simulink model "Dougherty1968_Linear"  (R2022b)
settings: Solver=VariableStepAuto  StartTime=0.0  StopTime=5000  RelTol=1e-3
model workspace (MAT data in the model file):
  Ix = 1000
  Iy = 1000
  Iz = 1000
  K_i = 1150
  K_p = 25
  T_c = 1
  frequency_multiplier = 10000
  h = 150
  k_phi = 50
  offset = 0.611
  omega_0 = 0.000727
  phi_0 = 0.0175
  phi_dot_0 = 0
  psi_0 = 0
  psi_dot_0 = 0
  tau = 25
libraries: simulink x2
settings Model: Creator=Kirtan  LastModifiedBy=Kirtan

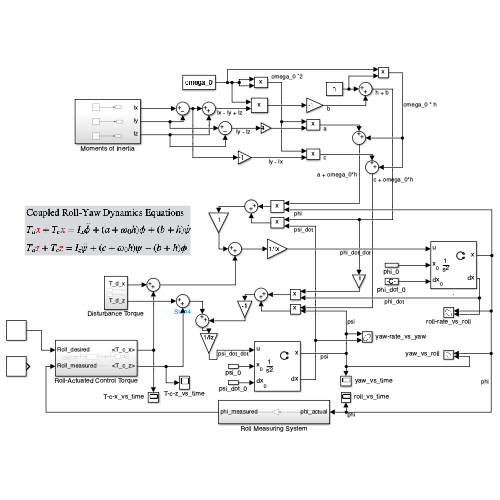
[thumbnail: Simulink's stored preview of the top-level diagram]
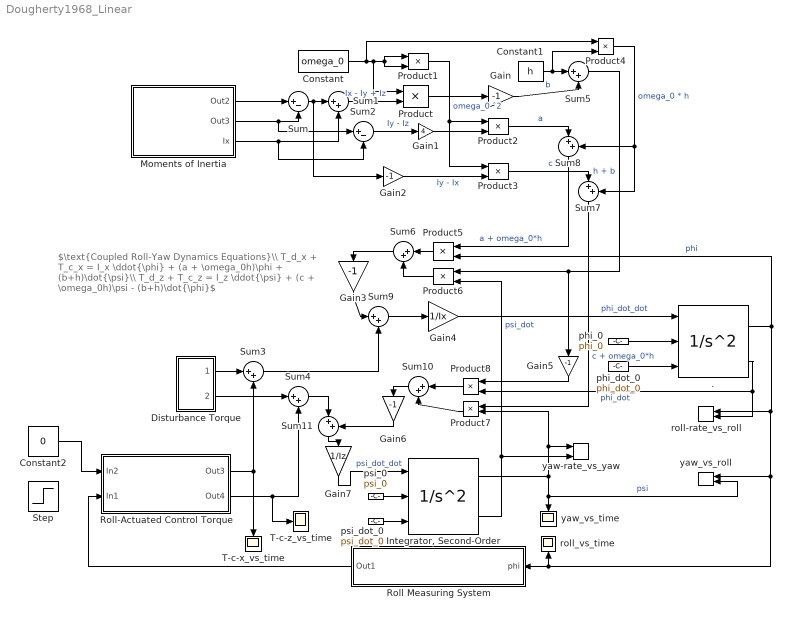
== system Dougherty1968_Linear ==
  note: $\text{Coupled Roll-Yaw Dynamics Equations}\\ T_d_x + T_c_x = I_x \ddot{\phi} + (a + \omega_0h)\phi + (b+h)\dot{\psi}\\ T_d_z + T_c_z = I_z \ddot{\psi} + (c + \omega_0h)\psi - (b+h)\dot{\phi}$
  . : SecondOrderIntegrator  ICSourceX=external  ICX=0.0175  WrapX=on  ICSourceDXDT=external
  Constant : Constant  Value=omega_0
  Constant1 : Constant  Value=h
  Constant2 : Constant  Value=0
  Disturbance Torque : Subsystem
  Gain{,2..3,5..6} (5 alike) : Gain  Gain=-1
  Gain1 : Gain  Gain=4
  Gain4 : Gain  Gain=1/Ix
  Gain7 : Gain  Gain=1/Iz
  "Integrator, Second-Order" : SecondOrderIntegrator  ICSourceX=external  ICX=0  WrapX=on  ICSourceDXDT=external
  Moments of Inertia : Subsystem
  Product{,1..8} (9 alike) : Product
  Roll Measuring System : Subsystem
  Roll-Actuated Control Torque : Subsystem
  Step : Step  After=0.5  SampleTime=0
  Sum : Sum  Inputs=|+-
  Sum{1,3..11} (10 alike) : Sum  Inputs=|++
  Sum2 : Sum  Inputs=|+-
  T-c-x_vs_time : Scope
  T-c-z_vs_time : Scope
  phi_0 : Constant  Value=phi_0
  phi_dot_0 : Constant  Value=phi_dot_0
  psi_0 : Constant  Value=psi_0
  psi_dot_0 : Constant  Value=psi_dot_0
  roll-rate_vs_roll : Record  FileSettingsInternal="{\"entries\":[{\"content\":{\"excelSettings\":{\"content\":{},\"type\":\"Streamout.ExcelSettings\"}},\"type\":\"Streamout.FileSettingStorage\",\"uuid\":\"38b1782c-b750-4221-bec9-1b26ef69e43c\"}],\"packageUris\":[\"http://schema.mathworks.com/mf0/streamout_blocks/R2020a\"],\"version\":\"1.0\"}"  Layout=[1 1]  SignalsInternal="{\"entries\":[{\"content\":{\"signals\":[{\"content\":{\"blockPath\":[\"Dougherty1968_Linear/roll-rate_vs_roll\"],\"channel\":[],\"dimensions\":[1],\"domain\":\"Dougherty1968_Linear/roll-rate_vs_roll\",\"lineColor\":\"#a2142f\",\"plots\":[],\"port\":1,\"sid\":[\"\"],\"signalID\":3010,\"signalName\":\"phi\"},\"type\":\"RecordBlkView.Signal\",\"uuid\":\"febe00e5-6828-4057-a697-2c8ae211d2fd\"},{\"content\":{\"blockPath\":[\"Dougherty1968_Linear/roll-rate_vs_roll\"],\"channel\":[],\"dimensions\":[1],\"domain\":\"Dougherty1968_Linear/roll-rate_vs_roll\",\"lineColor\":\"#139fff\",\"plots\":[],\"port\":2,\"sid\":[\"\"],\"signalID\":3014,\"signalName\":\"phi_dot\"},\"type\":\"RecordBlkView.Signal\",\"uuid\":\"0362f5a0-9189-4508-a90b-fc9b0aa5cd35\"}]},\"type\":\"RecordBlkView.InputSignals\",\"uuid\":\"35eba2d3-5ff9-4292-a791-673992ec5498\"}],\"packageUris\":[\"http://schema.mathworks.com/mf0/streamout_blocks/R2020a\"],\"version\":\"1.0\"}"  VisualizationBindings="{\"xyplotplugin\":{\"info\":[{\"series\":[{\"bindingParametersList\":[{\"parameter\":\"X-Axis\",\"signalID\":2664,\"signalName\":\"phi\"},{\"parameter\":\"Y-Axis\",\"signalID\":2668,\"signalName\":\"phi_dot\"}],\"seriesID\":41671}],\"subplotID\":1}]}}"  CompatibilityTag=XY
  roll_vs_time : Scope
  yaw-rate_vs_yaw : Record  FileSettingsInternal="{\"entries\":[{\"content\":{\"excelSettings\":{\"content\":{},\"type\":\"Streamout.ExcelSettings\"}},\"type\":\"Streamout.FileSettingStorage\",\"uuid\":\"572d4451-93c2-4438-9212-4a7969988a5a\"}],\"packageUris\":[\"http://schema.mathworks.com/mf0/streamout_blocks/R2020a\"],\"version\":\"1.0\"}"  Layout=[1 1]  SignalsInternal="{\"entries\":[{\"content\":{\"signals\":[{\"content\":{\"blockPath\":[\"Dougherty1968_Linear/yaw-rate_vs_yaw\"],\"channel\":[],\"dimensions\":[1],\"domain\":\"Dougherty1968_Linear/yaw-rate_vs_yaw\",\"lineColor\":\"#ff6929\",\"plots\":[],\"port\":1,\"sid\":[\"\"],\"signalID\":3018,\"signalName\":\"psi\"},\"type\":\"RecordBlkView.Signal\",\"uuid\":\"c75b039f-e5b5-43bc-a5bd-d29f9eaa01d0\"},{\"content\":{\"blockPath\":[\"Dougherty1968_Linear/yaw-rate_vs_yaw\"],\"channel\":[],\"dimensions\":[1],\"domain\":\"Dougherty1968_Linear/yaw-rate_vs_yaw\",\"lineColor\":\"#b746ff\",\"plots\":[],\"port\":2,\"sid\":[\"\"],\"signalID\":3022,\"signalName\":\"psi_dot\"},\"type\":\"RecordBlkView.Signal\",\"uuid\":\"d12e7a4e-fcf9-48c9-99a7-346f6f1f2049\"}]},\"type\":\"RecordBlkView.InputSignals\",\"uuid\":\"9e26259a-e0ce-410a-a403-7f15970c20ca\"}],\"packageUris\":[\"http://schema.mathworks.com/mf0/streamout_blocks/R2020a\"],\"version\":\"1.0\"}"  VisualizationBindings="{\"xyplotplugin\":{\"info\":[{\"series\":[{\"bindingParametersList\":[{\"parameter\":\"X-Axis\",\"signalID\":2672,\"signalName\":\"psi\"},{\"parameter\":\"Y-Axis\",\"signalID\":2676,\"signalName\":\"psi_dot\"}],\"seriesID\":11210}],\"subplotID\":1}]}}"  CompatibilityTag=XY
  yaw_vs_roll : Record  FileSettingsInternal="{\"entries\":[{\"content\":{\"excelSettings\":{\"content\":{},\"type\":\"Streamout.ExcelSettings\"}},\"type\":\"Streamout.FileSettingStorage\",\"uuid\":\"d29fa0e4-8fd2-49bc-bd02-98035cecc01b\"}],\"packageUris\":[\"http://schema.mathworks.com/mf0/streamout_blocks/R2020a\"],\"version\":\"1.0\"}"  Layout=[1 1]  SignalsInternal="{\"entries\":[{\"content\":{\"signals\":[{\"content\":{\"blockPath\":[\"Dougherty1968_Linear/yaw_vs_roll\"],\"channel\":[],\"dimensions\":[1],\"domain\":\"Dougherty1968_Linear/yaw_vs_roll\",\"lineColor\":\"#64d413\",\"plots\":[],\"port\":1,\"sid\":[\"\"],\"signalID\":3026,\"signalName\":\"phi\"},\"type\":\"RecordBlkView.Signal\",\"uuid\":\"2368424b-8444-41ae-ac92-b649c9339808\"},{\"content\":{\"blockPath\":[\"Dougherty1968_Linear/yaw_vs_roll\"],\"channel\":[],\"dimensions\":[1],\"domain\":\"Dougherty1968_Linear/yaw_vs_roll\",\"lineColor\":\"#ff13a6\",\"plots\":[],\"port\":2,\"sid\":[\"\"],\"signalID\":3030,\"signalName\":\"psi\"},\"type\":\"RecordBlkView.Signal\",\"uuid\":\"983d903b-1049-4754-85d1-0d6e5346058d\"}]},\"type\":\"RecordBlkView.InputSignals\",\"uuid\":\"64582cca-b1eb-4e4a-b771-a2ba1b9482e3\"}],\"packageUris\":[\"http://schema.mathworks.com/mf0/streamout_blocks/R2020a\"],\"version\":\"1.0\"}"  VisualizationBindings="{\"xyplotplugin\":{\"info\":[{\"series\":[{\"bindingParametersList\":[{\"parameter\":\"X-Axis\",\"signalID\":2680,\"signalName\":\"phi\"},{\"parameter\":\"Y-Axis\",\"signalID\":2684,\"signalName\":\"psi\"}],\"seriesID\":53193}],\"subplotID\":1}]}}"  CompatibilityTag=XY
  yaw_vs_time : Scope
  wires:
  ./2 -> roll-rate_vs_roll/2, Product8/2  "phi_dot"
  ./1 -> Product5/2, roll-rate_vs_roll/1, roll_vs_time/1, Roll Measuring System/1(phi), yaw_vs_roll/1  "phi"
  Gain4/1 -> ./1  "phi_dot_dot"
  "Integrator, Second-Order"/2 -> Product6/2, yaw-rate_vs_yaw/2  "psi_dot"
  "Integrator, Second-Order"/1 -> yaw_vs_time/1, yaw_vs_roll/2, yaw-rate_vs_yaw/1, Product7/2  "psi"
  Gain7/1 -> "Integrator, Second-Order"/1  "psi_dot_dot"
  Moments of Inertia/1(Out2) -> Sum/1
  Moments of Inertia/2(Out3) -> Sum2/1, Sum/2
  Sum/1 -> Gain2/1, Sum1/1
  Moments of Inertia/3(Ix) -> Sum2/2, Sum1/2
  Constant/1 -> Product4/1, Product1/2, Product1/1, Product/1
  Sum1/1 -> Product/2  "Ix - Iy + Iz"
  Product/1 -> Gain/1
  Sum2/1 -> Gain1/1  "Iy - Iz"
  Gain/1 -> Sum5/2  "b"
  Product1/1 -> Product3/1, Product2/1  "omega_0 ˆ2"
  Gain1/1 -> Product2/2
  Product2/1 -> Sum8/1  "a"
  Gain2/1 -> Product3/2  "Iy - Ix"
  Product3/1 -> Sum7/1  "c"
  Disturbance Torque/1(Out1) -> Sum3/1
  Roll-Actuated Control Torque/1(Out3) -> Sum3/2, T-c-x_vs_time/1
  Disturbance Torque/2(Out2) -> Sum4/1
  Roll-Actuated Control Torque/2(Out4) -> T-c-z_vs_time/1, Sum4/2
  Constant1/1 -> Product4/2, Sum5/1
  Sum5/1 -> Product6/1, Gain5/1  "h + b"
  Product4/1 -> Sum7/2, Sum8/2  "omega_0 * h"
  Sum7/1 -> Product7/1  "c + omega_0*h"
  Sum8/1 -> Product5/1  "a + omega_0*h"
  Product5/1 -> Sum6/1
  Product6/1 -> Sum6/2
  Sum6/1 -> Gain3/1
  Sum3/1 -> Sum9/2
  Gain3/1 -> Sum9/1
  Sum9/1 -> Gain4/1
  Product7/1 -> Sum10/2
  Gain5/1 -> Product8/1
  Sum10/1 -> Gain6/1
  Product8/1 -> Sum10/1
  Sum4/1 -> Sum11/1
  Gain6/1 -> Sum11/2
  Sum11/1 -> Gain7/1
  Roll Measuring System/1(Out1) -> Roll-Actuated Control Torque/2(In1)
  Constant2/1 -> Roll-Actuated Control Torque/1(In2)
  psi_0/1 -> "Integrator, Second-Order"/2
  phi_0/1 -> ./2
  phi_dot_0/1 -> ./3
  psi_dot_0/1 -> "Integrator, Second-Order"/3

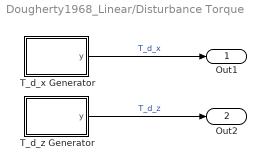
== system Dougherty1968_Linear/Disturbance Torque ==
  T_d_x Generator : Subsystem
  T_d_z Generator : Subsystem
  Out1 : Outport
  Out2 : Outport  Port=2
  wires:
  T_d_z Generator/1(y) -> Out2/1  "T_d_z"
  T_d_x Generator/1(y) -> Out1/1  "T_d_x"

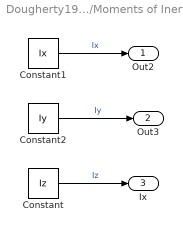
== system Dougherty1968_Linear/Moments of Inertia ==
  Constant : Constant  Value=Iz
  Constant1 : Constant  Value=Ix
  Constant2 : Constant  Value=Iy
  Out2 : Outport
  Out3 : Outport  Port=2
  Ix : Outport  Port=3
  wires:
  Constant/1 -> Ix/1  "Iz"
  Constant1/1 -> Out2/1  "Ix"
  Constant2/1 -> Out3/1  "Iy"

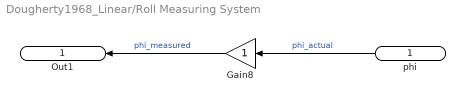
== system Dougherty1968_Linear/Roll Measuring System ==
  phi : Inport
  Gain8 : Gain
  Out1 : Outport
  wires:
  Gain8/1 -> Out1/1  "phi_measured"
  phi/1 -> Gain8/1  "phi_actual"

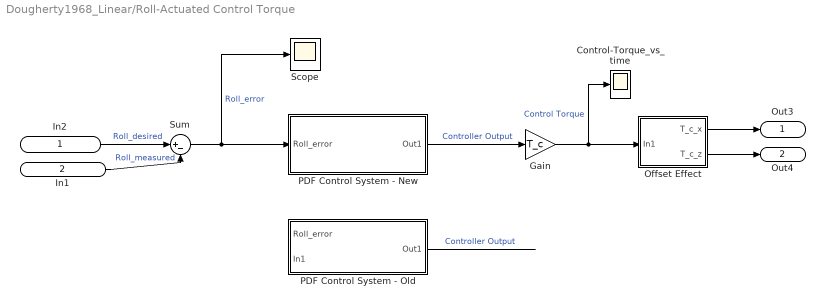
== system Dougherty1968_Linear/Roll-Actuated Control Torque ==
  In2 : Inport
  In1 : Inport  Port=2
  Control-Torque_vs_time : Scope
  Gain : Gain  Gain=T_c
  Offset Effect : Subsystem
  PDF Control System - New : Subsystem
  PDF Control System - Old : Subsystem
  Scope : Scope
  Sum : Sum  Inputs=|+-
  Out3 : Outport
  Out4 : Outport  Port=2
  wires:
  In1/1 -> Sum/2  "Roll_measured"
  In2/1 -> Sum/1  "Roll_desired"
  PDF Control System - Old/1(Out1) -> ?  "Controller Output"
  Sum/1 -> PDF Control System - New/1(Roll_error), Scope/1  "Roll_error"
  Gain/1 -> Control-Torque_vs_time/1, Offset Effect/1(In1)  "Control Torque"
  Offset Effect/1(T_c_x) -> Out3/1
  Offset Effect/2(T_c_z) -> Out4/1
  ? -> PDF Control System - Old/1(Roll_error)
  ? -> PDF Control System - Old/2(In1)
  PDF Control System - New/1(Out1) -> Gain/1  "Controller Output"

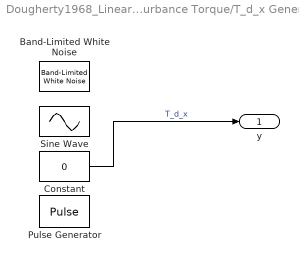
== system Dougherty1968_Linear/Disturbance Torque/T_d_x Generator ==
  Band-Limited White Noise : simulink/Sources/Band-Limited White Noise  Cov=[0.1]  Ts=0.1  seed=[23341]
  Constant : Constant  Value=0
  Pulse Generator : DiscretePulseGenerator  PulseType=Time based  Period=10  PulseWidth=5
  Sine Wave : Sin  Amplitude=0.005  Frequency=0.005  SampleTime=0
  y : Outport
  wires:
  Constant/1 -> y/1  "T_d_x"

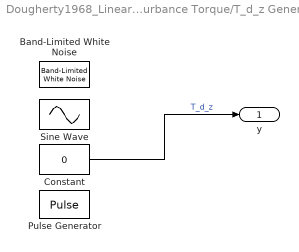
== system Dougherty1968_Linear/Disturbance Torque/T_d_z Generator ==
  Band-Limited White Noise : simulink/Sources/Band-Limited White Noise  Cov=[0.1]  Ts=0.1  seed=[23341]
  Constant : Constant  Value=0
  Pulse Generator : DiscretePulseGenerator  PulseType=Time based  Period=10  PulseWidth=5
  Sine Wave : Sin  Amplitude=0.005  Frequency=0.005  SampleTime=0
  y : Outport
  wires:
  Constant/1 -> y/1  "T_d_z"

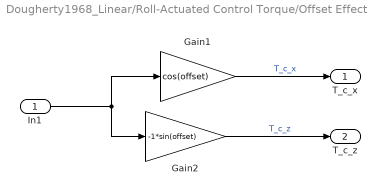
== system Dougherty1968_Linear/Roll-Actuated Control Torque/Offset Effect ==
  In1 : Inport
  Gain1 : Gain  Gain=cos(offset)
  Gain2 : Gain  Gain=-1*sin(offset)
  T_c_x : Outport
  T_c_z : Outport  Port=2
  wires:
  Gain2/1 -> T_c_z/1  "T_c_z"
  Gain1/1 -> T_c_x/1  "T_c_x"
  In1/1 -> Gain2/1, Gain1/1

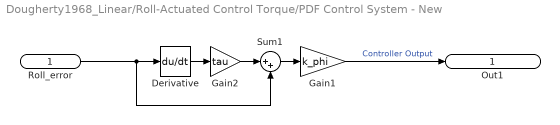
== system Dougherty1968_Linear/Roll-Actuated Control Torque/PDF Control System - New ==
  Roll_error : Inport
  Derivative : Derivative
  Gain1 : Gain  Gain=k_phi
  Gain2 : Gain  Gain=tau
  Sum1 : Sum  Inputs=|++
  Out1 : Outport
  wires:
  Gain2/1 -> Sum1/1
  Roll_error/1 -> Sum1/2, Derivative/1
  Derivative/1 -> Gain2/1
  Gain1/1 -> Out1/1  "Controller Output"
  Sum1/1 -> Gain1/1

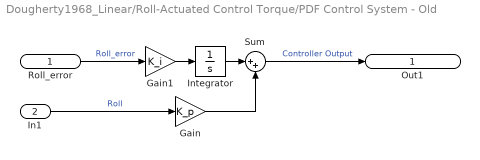
== system Dougherty1968_Linear/Roll-Actuated Control Torque/PDF Control System - Old ==
  Roll_error : Inport
  In1 : Inport  Port=2
  Gain : Gain  Gain=K_p
  Gain1 : Gain  Gain=K_i
  Integrator : Integrator
  Sum : Sum  Inputs=|++
  Out1 : Outport
  wires:
  Sum/1 -> Out1/1  "Controller Output"
  Roll_error/1 -> Gain1/1  "Roll_error"
  In1/1 -> Gain/1  "Roll"
  Gain/1 -> Sum/2
  Gain1/1 -> Integrator/1
  Integrator/1 -> Sum/1
